simulink model "levitador"  (R2023b)
settings: Solver=ode45  StartTime=0.0  StopTime=0.5  MaxStep=1e-3  RelTol=1e-3
values from neighbouring files (symbols this model uses):
  AL = double(subs(A_par))    [modeloMatematico.m]    (also in motor copy.m = double(subs(A,{x1,x2,x3,Vin,R,L,Ki,Kv,Jm,Jl,Bm,Bl,n,g,d,m},{; motor.m = double(subs(A,{x1,x2,x3,Vin,R,L,Ki,Kv,Jm,Jl,Bm,Bl,n,g,d,m},{; untitled.m = double(subs(A,{x1,x2,x3,u,M,g,R,L},{x10n,x20n,x30n,u0n,Mo,go)
  BL = double(subs(B_par))    [modeloMatematico.m]    (also in motor copy.m = double(subs(B,{x1,x2,x3,Vin,R,L,Ki,Kv,Jm,Jl,Bm,Bl,n,g,d,m},{; motor.m = double(subs(B,{x1,x2,x3,Vin,R,L,Ki,Kv,Jm,Jl,Bm,Bl,n,g,d,m},{; untitled.m = double(subs(B,{x1,x2,x3,u,M,g,R,L},{x10n,x20n,x30n,u0n,Mo,go)
  CL = double(subs(C_par))    [modeloMatematico.m]    (also in motor copy.m = [0 0 1/n0]; motor.m = [0 0 1/n0]; untitled.m = double(subs(C,{x1,x2,x3,u,M,g,R,L},{x10n,x20n,x30n,u0n,Mo,go)
  go = 9.81    [untitled.m]
  Lo = 0.7    [untitled.m]
  Mo = 0.2    [untitled.m]
  Ro = 8    [untitled.m]
  u0n = x30n*Ro    [untitled.m]
  x10n = 0.1    [untitled.m]
  x20n = 0    [untitled.m]
  x30n = sqrt(Mo*go*x10n)    [untitled.m]
settings Model: Creator=salones  LastModifiedBy=salones

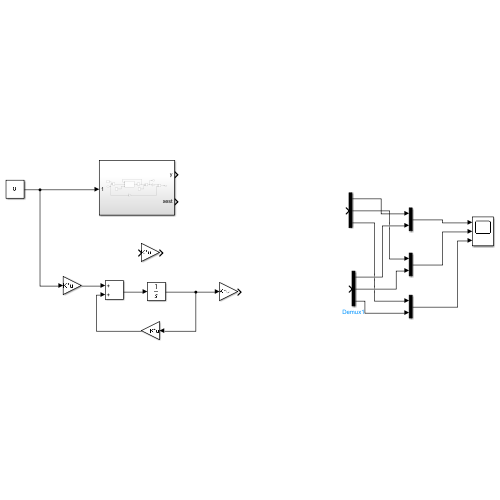
[thumbnail: Simulink's stored preview of the top-level diagram]
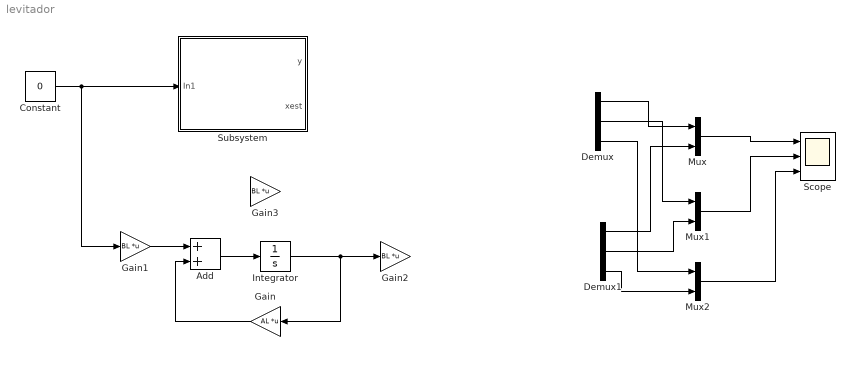
== system levitador ==
  Add : Sum
  Constant : Constant  Value=0
  Demux : Demux  Outputs=3
  Demux1 : Demux  Outputs=3
  Gain : Gain  Gain=AL  Multiplication=Matrix(K*u)
  Gain1 : Gain  Gain=BL  Multiplication=Matrix(K*u)
  Gain2 : Gain  Gain=BL  Multiplication=Matrix(K*u)
  Gain3 : Gain  Gain=BL  Multiplication=Matrix(K*u)
  Integrator : Integrator
  Mux : Mux  Inputs=2
  Mux1 : Mux  Inputs=2
  Mux2 : Mux  Inputs=2
  Scope : Scope  NumInputPorts=3
  Subsystem : Subsystem
  wires:
  Constant/1 -> Gain1/1, Subsystem/1(In1)
  Gain1/1 -> Add/1
  Add/1 -> Integrator/1
  Gain/1 -> Add/2
  Integrator/1 -> Gain2/1, Gain/1
  Demux/1 -> Mux/1
  Demux1/1 -> Mux/2
  Mux/1 -> Scope/1
  Demux/2 -> Mux1/1
  Demux1/2 -> Mux1/2
  Demux/3 -> Mux2/1
  Demux1/3 -> Mux2/2
  Mux1/1 -> Scope/2
  Mux2/1 -> Scope/3

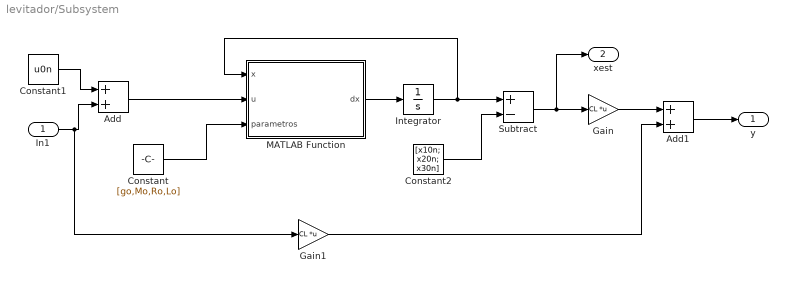
== system levitador/Subsystem ==
  In1 : Inport
  Add : Sum
  Add1 : Sum
  Constant : Constant  Value=[go,Mo,Ro,Lo]
  Constant1 : Constant  Value=u0n
  Constant2 : Constant  Value=[x10n; x20n; x30n]
  Gain : Gain  Gain=CL  Multiplication=Matrix(K*u)
  Gain1 : Gain  Gain=CL  Multiplication=Matrix(K*u)
  Integrator : Integrator  InitialCondition=[x10n; x20n; x30n]
  MATLAB Function : MATLAB Function  TreatAsAtomicUnit=on
  Subtract : Sum  Inputs=+-
  y : Outport
  xest : Outport  Port=2
  wires:
  Integrator/1 -> Subtract/1, MATLAB Function/1(x)
  Constant/1 -> MATLAB Function/3(parametros)
  In1/1 -> Gain1/1, Add/2
  Constant1/1 -> Add/1
  Constant2/1 -> Subtract/2
  MATLAB Function/1(dx) -> Integrator/1
  Add/1 -> MATLAB Function/2(u)
  Subtract/1 -> xest/1, Gain/1
  Gain/1 -> Add1/1
  Gain1/1 -> Add1/2
  Add1/1 -> y/1

== matlab function levitador/Subsystem/MATLAB Function ==
  data: x input; u input; dx output; parametros input
function dx = fcn(x,u,parametros)

x1 = x(1);
x2 = x(2);
x3 = x(3);
g = parametros(1);
M = parametros(2);
R = parametros(3);
L = parametros(4);

f1 = x2;
f2 = g - x3^2/(M*x1);
f3 = -R*x3/L + u/L;
dx = [f1; f2; f3];
